simulink model "Single_motor_flyer_controller_2017b"  (R2017b)
settings: Solver=VariableStepAuto  StartTime=0.0  StopTime=10.0  RelTol=1e-3
libraries: vrlib x1
settings Model: Creator=WEIDONG  LastModifiedBy=WEIDONG

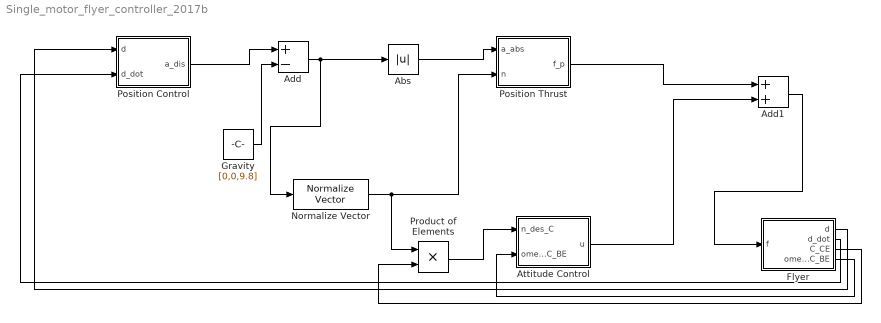
== system Single_motor_flyer_controller_2017b ==
  " Attitude Control" : MATLAB Function  TreatAsAtomicUnit=on
  Abs : Abs
  Add : Sum  Inputs=+-
  Add1 : Sum
  Flyer : MATLAB Function  TreatAsAtomicUnit=on
  Gravity : Constant  Value=[0,0,9.8]
  Normalize Vector : vrlib/Utilities/Normalize Vector  maxzero=0
      settings: SourceProductName=Simulink 3D Animation  SourceProductBaseCode=VR
  Position Control : MATLAB Function  TreatAsAtomicUnit=on
  Position Thrust : MATLAB Function  TreatAsAtomicUnit=on
  Product of Elements : Product
  wires:
  Position Control/1(a_dis) -> Add/1
  Flyer/2(d_dot) -> Position Control/2(d_dot)
  Gravity/1 -> Add/2
  Add/1 -> Normalize Vector/1, Abs/1
  Abs/1 -> Position Thrust/1(a_abs)
  Normalize Vector/1 -> Product of Elements/1, Position Thrust/2(n)
  Flyer/3(C_CE) -> Product of Elements/2
  Product of Elements/1 -> " Attitude Control"/1(n_des_C)
  Position Thrust/1(f_p) -> Add1/1
  " Attitude Control"/1(u) -> Add1/2
  Add1/1 -> Flyer/1(f)
  Flyer/1(d) -> Position Control/1(d)
  Flyer/4(omega_C_BE) -> " Attitude Control"/2(omega_C_BE)

== matlab function Single_motor_flyer_controller_2017b/Position Control ==
  data: d input; a_dis output; d_dot input
function a_dis = fcn(d,d_dot)
epsilon=1;
omega=1;
a_dis = -2*epsilon*omega*d_dot-omega^2*d;

== matlab function Single_motor_flyer_controller_2017b/Position Thrust ==
  data: a_abs input; f_p output; n input
function f_p = fcn(a_abs, n)
z_B=[0,0,1];
m=0.217;

f_p = a_abs*m/dot(z_B,n);

== matlab function Single_motor_flyer_controller_2017b/ Attitude Control ==
  data: n_des_C input; u output; omega_C_BE input
function u = fcn(n_des_C,omega_C_BE)


u = 1;

== matlab function Single_motor_flyer_controller_2017b/Flyer ==
  data: f input; d output; d_dot output; C_CE output; omega_C_BE output
function [d,d_dot,C_CE,omega_C_BE] = fcn(f)

d = 0;
d_dot=0;
C_CE=0;
omega_C_BE=0;
